simulink library "ActivationContainerCommented"  (R2017b)
settings: Solver=VariableStepAuto  StartTime=0.0  StopTime=10.0  RelTol=1e-3
undefined symbols (not defined in the file): Subsystem0
settings Model: Creator=Beni  LastModifiedBy=Beni

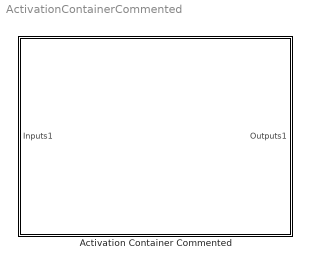
== system ActivationContainerCommented ==
  Activation Container Commented : Subsystem  mask(BlockActivationEnabled){Status0=Active, Subsystem0=Subsystem0, Status1=Inactive, Subsystem1=, Status2=Inactive, Subsystem2=, Status3=Inactive, Subsystem3=, Status4=Inactive, Subsystem4=, Status5=Inactive, Subsystem5=, Status6=Inactive, Subsystem6=, Status7=Inactive, Subsystem7=, Status8=Inactive, Subsystem8=, Status9=Inactive, Subsystem9=}
      mask prompts: Status0 "Activity status of "Subsystem0":"; Subsystem0 "Invisible Help Variable"; Status1 "Activity status of "Subsystem1":"; Subsystem1 "Invisible Help Variable"; Status2 "Activity status of "Subsystem2":"; Subsystem2 "Invisible Help Variable"; Status3 "Activity status of "Test3":"; Subsystem3 "Invisible Help Variable"; Status4 "Activity status of "Enabled Subsystem4":"; Subsystem4 "Invisible Help Variable"; Status5 "Activity status of "Enabled Subsystem5":"; Subsystem5 "Invisible Help Variable"; Status6 "Activity status of "Enabled Subsystem6":"; Subsystem6 "Invisible Help Variable"; Status7 "Activity status of "Enabled Subsystem7" [-]:"; Subsystem7 "Invisible Help Variable"; Status8 "Activity status of "Enabled Subsystem8" [-]:"; Subsystem8 "Invisible Help Variable"; Status9 "Activity status of "Enabled Subsystem9" [-]:"; Subsystem9 "Invisible Help Variable"
      mask help:
      | <Author> Benedikt Taiber </Author>
      | <Date> 25/09/2018 </Date>
      |
      | <Description>
      | This block can contain up to ten subsystems, that can be activated or deactivated for the simulation, depending on the user's input within the mask dialog. New subsystems can be added or already existing subsystems deleted by clicking the corresponding buttons on the mask dialog. The subsystems can also be de-/activated programmatically by setting the parameter "StatusX" to the corresponding "SubsystemX" to " 'Active/Inactive' ".
      | </Description>
      mask init:
      | Init_ActivationContainer_Commented();
      settings: OpenFcn=|
      | set_param(gcb,'LinkStatus','none');
      | Init_ActivationContainer_Commented();
      | open_system(gcb,'mask');
      mask Help:
      | <Parameters>
      | Activity status of "EnabledSubsystemX" [-]:
      | 	<Active, Inactive>
      | </Parameters>
      | 
      | <Inputs>
      | Depending on content of subsystem
      | </Inputs>
      | 
      | <Outputs>
      | Depending on content of subsystem
      | </Outputs>
      mask TypeOptions Status0: Active | Inactive
      mask Callback Status0:
      | if strcmp(get_param(gcb,'Status0'),'Active') && ~isempty(get_param(gcb,'Subsystem0'))
      |     set_param([gcb '/' get_param(gcb,'Subsystem0')],'Commented','Off');
      | elseif strcmp(get_param(gcb,'Status0'),'Inactive') && ~isempty(get_param(gcb,'Subsystem0'))
      |     set_param([gcb '/' get_param(gcb,'Subsystem0')],'Commented','On');
      | end
      mask TypeOptions Status1: Active | Inactive
      mask Callback Status1:
      | if strcmp(get_param(gcb,'Status1'),'Active') && ~isempty(get_param(gcb,'Subsystem1'))
      |     set_param([gcb '/' get_param(gcb,'Subsystem1')],'Commented','Off');
      | elseif strcmp(get_param(gcb,'Status1'),'Inactive') && ~isempty(get_param(gcb,'Subsystem1'))
      |     set_param([gcb '/' get_param(gcb,'Subsystem1')],'Commented','On');
      | end
      mask TypeOptions Status2: Active | Inactive
      mask Callback Status2:
      | if strcmp(get_param(gcb,'Status2'),'Active') && ~isempty(get_param(gcb,'Subsystem2'))
      |     set_param([gcb '/' get_param(gcb,'Subsystem2')],'Commented','Off');
      | elseif strcmp(get_param(gcb,'Status2'),'Inactive') && ~isempty(get_param(gcb,'Subsystem2'))
      |     set_param([gcb '/' get_param(gcb,'Subsystem2')],'Commented','On');
      | end
      mask TypeOptions Status3: Active | Inactive
      mask Callback Status3:
      | if strcmp(get_param(gcb,'Status3'),'Active') && ~isempty(get_param(gcb,'Subsystem3'))
      |     set_param([gcb '/' get_param(gcb,'Subsystem3')],'Commented','Off');
      | elseif strcmp(get_param(gcb,'Status3'),'Inactive') && ~isempty(get_param(gcb,'Subsystem3'))
      |     set_param([gcb '/' get_param(gcb,'Subsystem3')],'Commented','On');
      | end
      mask TypeOptions Status4: Active | Inactive
      mask Callback Status4:
      | if strcmp(get_param(gcb,'Status4'),'Active') && ~isempty(get_param(gcb,'Subsystem4'))
      |     set_param([gcb '/' get_param(gcb,'Subsystem4')],'Commented','Off');
      | elseif strcmp(get_param(gcb,'Status4'),'Inactive') && ~isempty(get_param(gcb,'Subsystem4'))
      |     set_param([gcb '/' get_param(gcb,'Subsystem4')],'Commented','On');
      | end
      mask TypeOptions Status5: Active | Inactive
      mask Callback Status5:
      | if strcmp(get_param(gcb,'Status5'),'Active') && ~isempty(get_param(gcb,'Subsystem5'))
      |     set_param([gcb '/' get_param(gcb,'Subsystem5')],'Commented','Off');
      | elseif strcmp(get_param(gcb,'Status5'),'Inactive') && ~isempty(get_param(gcb,'Subsystem5'))
      |     set_param([gcb '/' get_param(gcb,'Subsystem5')],'Commented','On');
      | end
      mask TypeOptions Status6: Active | Inactive
      mask Callback Status6:
      | if strcmp(get_param(gcb,'Status6'),'Active') && ~isempty(get_param(gcb,'Subsystem6'))
      |     set_param([gcb '/' get_param(gcb,'Subsystem6')],'Commented','Off');
      | elseif strcmp(get_param(gcb,'Status6'),'Inactive') && ~isempty(get_param(gcb,'Subsystem6'))
      |     set_param([gcb '/' get_param(gcb,'Subsystem6')],'Commented','On');
      | end
      mask TypeOptions Status7: Active | Inactive
      mask Callback Status7:
      | if strcmp(get_param(gcb,'Status7'),'Active') && ~isempty(get_param(gcb,'Subsystem7'))
      |     set_param([gcb '/' get_param(gcb,'Subsystem7')],'Commented','Off');
      | elseif strcmp(get_param(gcb,'Status7'),'Inactive') && ~isempty(get_param(gcb,'Subsystem7'))
      |     set_param([gcb '/' get_param(gcb,'Subsystem7')],'Commented','On');
      | end
      mask TypeOptions Status8: Active | Inactive
      mask Callback Status8:
      | if strcmp(get_param(gcb,'Status8'),'Active') && ~isempty(get_param(gcb,'Subsystem8'))
      |     set_param([gcb '/' get_param(gcb,'Subsystem8')],'Commented','Off');
      | elseif strcmp(get_param(gcb,'Status8'),'Inactive') && ~isempty(get_param(gcb,'Subsystem8'))
      |     set_param([gcb '/' get_param(gcb,'Subsystem8')],'Commented','On');
      | end
      mask TypeOptions Status9: Active | Inactive
      mask Callback Status9:
      | if strcmp(get_param(gcb,'Status9'),'Active') && ~isempty(get_param(gcb,'Subsystem9'))
      |     set_param([gcb '/' get_param(gcb,'Subsystem9')],'Commented','Off');
      | elseif strcmp(get_param(gcb,'Status9'),'Inactive') && ~isempty(get_param(gcb,'Subsystem9'))
      |     set_param([gcb '/' get_param(gcb,'Subsystem9')],'Commented','On');
      | end
      mask DialogControl Container14 Prompt: Documentation:
      mask DialogControl Control14 Prompt: %<MaskHelp>
      mask DialogControl Container0 Prompt: Subsystem0 - "Status0":
      mask DialogControl Delete0 Prompt: Delete Subsystem
      mask DialogControl Delete0 Callback:
      | index = 0;
      | Delete_Button_Commented(index);
      | clear index
      mask DialogControl Container1 Prompt: Subsystem1 - "Status1":
      mask DialogControl Delete1 Prompt: Delete Subsystem
      mask DialogControl Delete1 Callback:
      | index = 1;
      | Delete_Button_Commented(index);
      | clear index;
      mask DialogControl Container2 Prompt: Subsystem2 - "Status2":
      mask DialogControl Delete2 Prompt: Delete Subsystem
      mask DialogControl Delete2 Callback:
      | index = 2;
      | Delete_Button_Commented(index);
      | clear index
      mask DialogControl Container3 Prompt: Subsystem3 - "Status3":
      mask DialogControl Delete3 Prompt: Delete Subsystem
      mask DialogControl Delete3 Callback:
      | index = 3;
      | Delete_Button_Commented(index);
      | clear index
      mask DialogControl Container4 Prompt: Subsystem4 - "Status4":
      mask DialogControl Delete4 Prompt: Delete Subsystem
      mask DialogControl Delete4 Callback:
      | index = 4;
      | Delete_Button_Commented(index);
      | clear index
      mask DialogControl Container5 Prompt: Subsystem5 - "Status5":
      mask DialogControl Delete5 Prompt: Delete Subsystem
      mask DialogControl Delete5 Callback:
      | index = 5;
      | Delete_Button_Commented(index);
      | clear index
      mask DialogControl Container6 Prompt: Subsystem6 - "Status6":
      mask DialogControl Delete6 Prompt: Delete Subsystem
      mask DialogControl Delete6 Callback:
      | index = 6;
      | Delete_Button_Commented(index);
      | clear index
      mask DialogControl Container7 Prompt: Subsystem7 - "Status7":
      mask DialogControl Delete7 Prompt: Delete Subsystem
      mask DialogControl Delete7 Callback:
      | index = 7;
      | Delete_Button_Commented(index);
      | clear index
      mask DialogControl Container8 Prompt: Subsystem8 - "Status8":
      mask DialogControl Delete8 Prompt: Delete Subsystem
      mask DialogControl Delete8 Callback:
      | index = 8;
      | Delete_Button_Commented(index);
      | clear index
      mask DialogControl Container9 Prompt: Subsystem9 - "Status9":
      mask DialogControl Delete9 Prompt: Delete Subsystem
      mask DialogControl Delete9 Callback:
      | index = 9;
      | Delete_Button_Commented(index);
      | clear index
      mask DialogControl ContainerControls Prompt: Controls:
      mask DialogControl new_system Prompt: Create new subsystem
      mask DialogControl new_system Callback:
      | New_Subsystem_Commented();
      | Init_ActivationContainer_Commented();
      mask DialogControl check_system Prompt: Look under mask
      mask DialogControl check_system Callback: open_system(gcb,'force')
      mask Display:
      | image('ContainerSymbol.jpg')
      |     %Show folder symbol on masked block

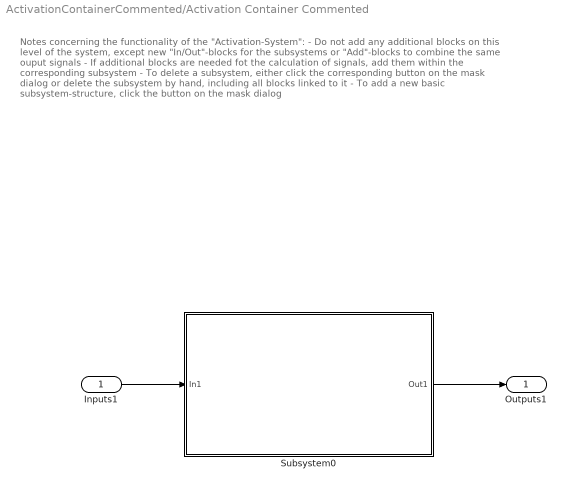
== system ActivationContainerCommented/Activation Container Commented ==
  note: Notes concerning the functionality of the "Activation-System":
      |
      | - Do not add any additional blocks on this level of the system, except new "In/Out"-blocks for
      |   the subsystems or "Add"-blocks to combine the same ouput signals
      | - If additional blocks are needed fot the calculation of signals, add them within the
      |   corresponding subsystem
      | - To delete a subsystem, either click the corresponding button on the mask dialog or delete
      |   the subsystem by hand, including all blocks linked to it
      | - To add a new basic subsystem-structure, click the button on the mask dialog
  Inputs1 : Inport
  Subsystem0 : Subsystem  Description=0
  Outputs1 : Outport
  wires:
  Inputs1/1 -> Subsystem0/1(In1)
  Subsystem0/1(Out1) -> Outputs1/1

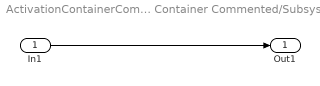
== system ActivationContainerCommented/Activation Container Commented/Subsystem0 ==
  In1 : Inport
  Out1 : Outport
  wires:
  In1/1 -> Out1/1
